simulink model "SGBMDisparity"  (R2021a)
settings: Solver=FixedStepDiscrete  StartTime=0.0  StopTime=simT  FixedStep=1  RelTol=1e-3
PreLoadFcn:
  | DL128 = Simulink.Variant('disparityLevels==128');
  | 
  | DLnot128 = Simulink.Variant('disparityLevels ~= 128');
  | 
  | disparityLevels = 64;
  | 
  | imgRowSize = 480;
  | 
  | imgColSize = 640;
  | 
  | P2 = 200; % Smoothness Penalty Large
  | P1 = 15;  % Smoothness Penalty Small
  | 
  | disparityFactor = 16;
  | 
  | uniquenessRatio = 5;
  | 
  | p = imgColSize - 1;
  | q = imgRowSize * imgColSize -1;
  | r = imgColSize - disparityLevels -1;
  | s = (imgRowSize*(imgColSize-disparityLevels))-1;
  | 
  | simT = 800*525
  | 
  | dtGain = 4;
InitFcn:
  | DL128 = Simulink.Variant('disparityLevels==128');
  | 
  | DLnot128 = Simulink.Variant('disparityLevels ~= 128');
  | 
  | img = imread(get_param('SGBMDisparity/stereoImage','FileName'));
  | 
  | [imgRowSize, imgColSize,chn] = size(img);
  | 
  | P2 = 200; % Smoothness Penalty Large
  | P1 = 15;  % Smoothness Penalty Small
  | 
  | disparityFactor = 16;
  | 
  | uniquenessRatio = str2num(get_param('SGBMDisparity/SGBMHDLAlgorithm/SGBMHDLAlgorithmWorker','UT'));
  | 
  | disparityLevels = str2num(get_param('SGBMDisparity/SGBMHDLAlgorithm/SGBMHDLAlgorithmWorker','DL'));
  | 
  | p = imgColSize - 1;
  | q = imgRowSize * imgColSize -1;
  | r = imgColSize - disparityLevels -1;
  | s = (imgRowSize*(imgColSize-disparityLevels))-1;
  | 
  | if imgRowSize == 720 && imgColSize == 1280
  | simT = 1650*750;
  | elseif imgRowSize == 540 && imgColSize == 960
  | simT = 1050*600;
  | elseif imgRowSize == 480 && imgColSize == 640
  | simT = 800*525;
  | end
  | 
  | %if imgRowSize == 720 && imgColSize == 1280
  | %dtGain = 2;
  | %elseif imgRowSize == 540 && imgColSize == 960
  | %dtGain = 2.6;
  | %elseif imgRowSize == 480 && imgColSize == 640
  | %dtGain = 4;
  | %end
  | 
  | dtGain = 8;
libraries: simulink x331, hdlsllib x113, visionhdlutilities x9, visionhdlio x2, visionsources x1
(part 3 of 6)

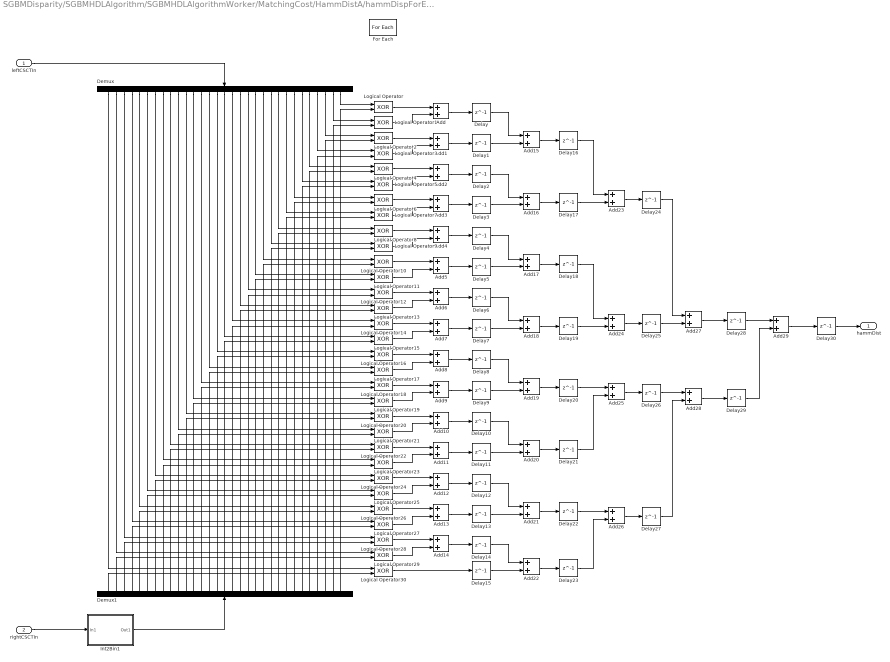
== system SGBMDisparity/SGBMHDLAlgorithm/SGBMHDLAlgorithmWorker/MatchingCost/HammDistA/hammDispForEach ==
  leftCSCTIn : Inport
  rightCSCTIn : Inport  Port=2  Partition=on  PartitionDimension=1  PartitionWidth=1  PartitionOffset=0
  Add{,1..14,22} (16 alike) : Sum  OutDataTypeStr=fixdt(0,2,0)
  Add{15..21,26} (8 alike) : Sum  OutDataTypeStr=fixdt(0,3,0)
  Add{23..25,28} (4 alike) : Sum  OutDataTypeStr=fixdt(0,4,0)
  Add27 : Sum  OutDataTypeStr=fixdt(0,5,0)
  Add29 : Sum  OutDataTypeStr=fixdt(0,5,0)
  Delay{,1..30} (31 alike) : Delay  DelayLength=1
  Demux : Demux  Outputs=31
  Demux1 : Demux  Outputs=31
  For Each : ForEach  DisableCoverage=on
  Int2Bin1 : Subsystem
  Logical Operator{,1..30} (31 alike) : Logic  Operator=XOR  OutDataTypeStr=boolean
  hammDist : Outport  ConcatenationDimension=1  VectorParamsAs1DForOutWhenUnconnected=off
  wires:
  Demux1/7 -> Logical Operator24/2
  Demux1/18 -> Logical Operator13/2
  Delay22/1 -> Add26/1
  Logical Operator19/1 -> Add9/2
  Demux/23 -> Logical Operator8/1
  Add26/1 -> Delay27/1
  Demux1/9 -> Logical Operator22/2
  Demux1/13 -> Logical Operator18/2
  Demux/10 -> Logical Operator21/1
  Demux/24 -> Logical Operator7/1
  Demux1/26 -> Logical Operator5/2
  Demux1/10 -> Logical Operator21/2
  Demux/14 -> Logical Operator17/1
  Demux1/17 -> Logical Operator14/2
  Delay18/1 -> Add24/1
  Demux1/15 -> Logical Operator16/2
  Demux1/11 -> Logical Operator20/2
  Demux/11 -> Logical Operator20/1
  Add27/1 -> Delay28/1
  Delay26/1 -> Add28/1
  Delay11/1 -> Add20/2
  Logical Operator13/1 -> Add6/2
  Add16/1 -> Delay17/1
  Add20/1 -> Delay21/1
  Demux/21 -> Logical Operator10/1
  Add18/1 -> Delay19/1
  Add23/1 -> Delay24/1
  Demux1/28 -> Logical Operator3/2
  Demux1/27 -> Logical Operator4/2
  Demux/26 -> Logical Operator5/1
  Demux/22 -> Logical Operator9/1
  Demux/25 -> Logical Operator6/1
  Demux/20 -> Logical Operator11/1
  Demux/8 -> Logical Operator23/1
  Demux1/29 -> Logical Operator2/2
  leftCSCTIn/1 -> Demux/1
  Logical Operator12/1 -> Add6/1
  Demux/19 -> Logical Operator12/1
  Add/1 -> Delay/1
  Demux/17 -> Logical Operator14/1
  Logical Operator22/1 -> Add11/1
  Demux/29 -> Logical Operator2/1
  Logical Operator16/1 -> Add8/1
  Logical Operator18/1 -> Add9/1
  Logical Operator17/1 -> Add8/2
  Logical Operator26/1 -> Add13/1
  Logical Operator24/1 -> Add12/1
  Logical Operator25/1 -> Add12/2
  Demux1/20 -> Logical Operator11/2
  Delay27/1 -> Add28/2
  Add13/1 -> Delay13/1
  Logical Operator4/1 -> Add2/1
  Logical Operator3/1 -> Add1/2
  Demux1/24 -> Logical Operator7/2
  Demux1/31 -> Logical Operator/2
  Logical Operator8/1 -> Add4/1
  Demux1/30 -> Logical Operator1/2
  Logical Operator5/1 -> Add2/2
  Logical Operator2/1 -> Add1/1
  Logical Operator7/1 -> Add3/2
  Logical Operator6/1 -> Add3/1
  Demux/30 -> Logical Operator1/1
  Delay29/1 -> Add29/2
  Demux1/25 -> Logical Operator6/2
  Logical Operator9/1 -> Add4/2
  Logical Operator14/1 -> Add7/1
  Demux/31 -> Logical Operator/1
  Delay21/1 -> Add25/2
  Delay24/1 -> Add27/1
  Delay23/1 -> Add26/2
  Logical Operator15/1 -> Add7/2
  Delay28/1 -> Add29/1
  Add28/1 -> Delay29/1
  Add22/1 -> Delay23/1
  Add25/1 -> Delay26/1
  Add24/1 -> Delay25/1
  Delay19/1 -> Add24/2
  Delay13/1 -> Add21/2
  rightCSCTIn/1 -> Int2Bin1/1(In1)
  Add1/1 -> Delay1/1
  Add17/1 -> Delay18/1
  Delay3/1 -> Add16/2
  Delay6/1 -> Add18/1
  Add12/1 -> Delay12/1
  Logical Operator30/1 -> Delay15/1
  Delay9/1 -> Add19/2
  Delay4/1 -> Add17/1
  Delay/1 -> Add15/1
  Add7/1 -> Delay7/1
  Add9/1 -> Delay9/1
  Add10/1 -> Delay10/1
  Add14/1 -> Delay14/1
  Add5/1 -> Delay5/1
  Add3/1 -> Delay3/1
  Logical Operator/1 -> Add/1
  Delay16/1 -> Add23/1
  Add29/1 -> Delay30/1
  Demux1/8 -> Logical Operator23/2
  Demux/4 -> Logical Operator27/1
  Demux1/5 -> Logical Operator26/2
  Demux/18 -> Logical Operator13/1
  Logical Operator1/1 -> Add/2
  Demux1/4 -> Logical Operator27/2
  Demux1/1 -> Logical Operator30/2
  Add2/1 -> Delay2/1
  Demux/16 -> Logical Operator15/1
  Demux1/12 -> Logical Operator19/2
  Demux1/2 -> Logical Operator29/2
  Delay12/1 -> Add21/1
  Demux/12 -> Logical Operator19/1
  Delay2/1 -> Add16/1
  Delay17/1 -> Add23/2
  Logical Operator27/1 -> Add13/2
  Delay20/1 -> Add25/1
  Demux/13 -> Logical Operator18/1
  Logical Operator28/1 -> Add14/1
  Add21/1 -> Delay22/1
  Demux/7 -> Logical Operator24/1
  Logical Operator21/1 -> Add10/2
  Demux/2 -> Logical Operator29/1
  Delay30/1 -> hammDist/1
  Demux1/19 -> Logical Operator12/2
  Delay15/1 -> Add22/2
  Demux/5 -> Logical Operator26/1
  Demux1/22 -> Logical Operator9/2
  Add6/1 -> Delay6/1
  Demux/28 -> Logical Operator3/1
  Delay7/1 -> Add18/2
  Logical Operator20/1 -> Add10/1
  Demux/6 -> Logical Operator25/1
  Logical Operator11/1 -> Add5/2
  Demux1/6 -> Logical Operator25/2
  Logical Operator23/1 -> Add11/2
  Add4/1 -> Delay4/1
  Delay8/1 -> Add19/1
  Add8/1 -> Delay8/1
  Add11/1 -> Delay11/1
  Demux/15 -> Logical Operator16/1
  Delay1/1 -> Add15/2
  Demux/9 -> Logical Operator22/1
  Demux/3 -> Logical Operator28/1
  Add15/1 -> Delay16/1
  Demux1/3 -> Logical Operator28/2
  Delay10/1 -> Add20/1
  Logical Operator29/1 -> Add14/2
  Demux1/23 -> Logical Operator8/2
  Delay14/1 -> Add22/1
  Delay5/1 -> Add17/2
  Demux1/21 -> Logical Operator10/2
  Demux/1 -> Logical Operator30/1
  Demux1/16 -> Logical Operator15/2
  Demux/27 -> Logical Operator4/1
  Demux1/14 -> Logical Operator17/2
  Add19/1 -> Delay20/1
  Logical Operator10/1 -> Add5/1
  Delay25/1 -> Add27/2
  Int2Bin1/1(Out1) -> Demux1/1

== system SGBMDisparity/SGBMHDLAlgorithm/SGBMHDLAlgorithmWorker/MatchingCost/HammDistA/pixelBusGenerator ==
  validIn : Inport
  Horizontal : hdlsllib/Sources/HDL Counter  CountType=Count limited  CountInit=0  CountStep=1  CountMax=hEnd  CountFromType=Initial value  CountFrom=0  CountResetPort=off  CountLoadPort=off  CountEnbPort=on  CountDirPort=off  CountHitOutputPort=off  CountDataType=Unsigned  CountWordLen=ceil(log2(hEnd))  CountFracLen=0  CountSampTime=1
  Logical Operator{3..6} (4 alike) : Logic  AllPortsSameDT=off  OutDataTypeStr=boolean
  Pixel Control Bus Creator : visionhdlutilities/Pixel Control Bus Creator
      settings: SourceProductBaseCode=VT
  Vertical : hdlsllib/Sources/HDL Counter  CountType=Count limited  CountInit=0  CountStep=1  CountMax=vEnd  CountFromType=Initial value  CountFrom=0  CountResetPort=off  CountLoadPort=off  CountEnbPort=on  CountDirPort=off  CountHitOutputPort=off  CountDataType=Unsigned  CountWordLen=ceil(log2(vEnd))  CountFracLen=0  CountSampTime=1
  hEnd : simulink/Logic and Bit Operations/Compare To Constant  relop===  const=hEnd  OutDataTypeStr=boolean
  hStart : simulink/Logic and Bit Operations/Compare To Constant  relop===  const=0  OutDataTypeStr=boolean
  vEnd : simulink/Logic and Bit Operations/Compare To Constant  relop===  const=vEnd  OutDataTypeStr=boolean
  vStart : simulink/Logic and Bit Operations/Compare To Constant  relop===  const=0  OutDataTypeStr=boolean
  busOut : Outport  VectorParamsAs1DForOutWhenUnconnected=off
  wires:
  validIn/1 -> Pixel Control Bus Creator/5, Vertical/1, Logical Operator4/1, Logical Operator5/1, Logical Operator6/1, Logical Operator3/1, Horizontal/1
  Horizontal/1 -> hEnd/1, hStart/1
  hEnd/1 -> Logical Operator4/2
  Vertical/1 -> vStart/1, vEnd/1
  vStart/1 -> Logical Operator5/2
  vEnd/1 -> Logical Operator6/2
  Logical Operator5/1 -> Pixel Control Bus Creator/3
  Logical Operator3/1 -> Pixel Control Bus Creator/1
  Logical Operator4/1 -> Pixel Control Bus Creator/2
  hStart/1 -> Logical Operator3/2
  Logical Operator6/1 -> Pixel Control Bus Creator/4
  Pixel Control Bus Creator/1 -> busOut/1

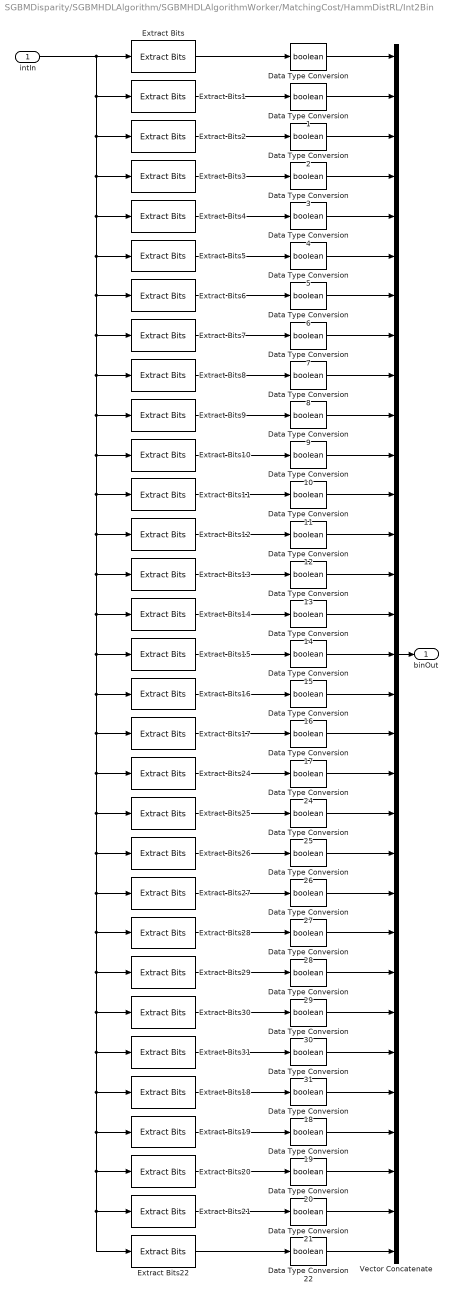
== system SGBMDisparity/SGBMHDLAlgorithm/SGBMHDLAlgorithmWorker/MatchingCost/HammDistRL/Int2Bin ==
  intIn : Inport
  Data Type Conversion{,1..22,24..31} (31 alike) : DataTypeConversion  OutDataTypeStr=boolean
  Extract Bits : simulink/Logic and Bit Operations/Extract Bits  bitsToExtract=Range of bits  numBits=8  bitIdxRange=[30]  outScalingMode=Treat bit field as an integer
  Extract Bits1 : simulink/Logic and Bit Operations/Extract Bits  bitsToExtract=Range of bits  numBits=8  bitIdxRange=[29]  outScalingMode=Treat bit field as an integer
  Extract Bits10 : simulink/Logic and Bit Operations/Extract Bits  bitsToExtract=Range of bits  numBits=8  bitIdxRange=[20]  outScalingMode=Preserve fixed-point scaling
  Extract Bits11 : simulink/Logic and Bit Operations/Extract Bits  bitsToExtract=Range of bits  numBits=8  bitIdxRange=[19]  outScalingMode=Preserve fixed-point scaling
  Extract Bits12 : simulink/Logic and Bit Operations/Extract Bits  bitsToExtract=Range of bits  numBits=8  bitIdxRange=[18]  outScalingMode=Preserve fixed-point scaling
  Extract Bits13 : simulink/Logic and Bit Operations/Extract Bits  bitsToExtract=Range of bits  numBits=8  bitIdxRange=[17]  outScalingMode=Preserve fixed-point scaling
  Extract Bits14 : simulink/Logic and Bit Operations/Extract Bits  bitsToExtract=Range of bits  numBits=8  bitIdxRange=[16]  outScalingMode=Preserve fixed-point scaling
  Extract Bits15 : simulink/Logic and Bit Operations/Extract Bits  bitsToExtract=Range of bits  numBits=8  bitIdxRange=[15]  outScalingMode=Preserve fixed-point scaling
  Extract Bits16 : simulink/Logic and Bit Operations/Extract Bits  bitsToExtract=Range of bits  numBits=8  bitIdxRange=[14]  outScalingMode=Preserve fixed-point scaling
  Extract Bits17 : simulink/Logic and Bit Operations/Extract Bits  bitsToExtract=Range of bits  numBits=8  bitIdxRange=[13]  outScalingMode=Preserve fixed-point scaling
  Extract Bits18 : simulink/Logic and Bit Operations/Extract Bits  bitsToExtract=Range of bits  numBits=8  bitIdxRange=[4]  outScalingMode=Preserve fixed-point scaling
  Extract Bits19 : simulink/Logic and Bit Operations/Extract Bits  bitsToExtract=Range of bits  numBits=8  bitIdxRange=[3]  outScalingMode=Preserve fixed-point scaling
  Extract Bits2 : simulink/Logic and Bit Operations/Extract Bits  bitsToExtract=Range of bits  numBits=8  bitIdxRange=[28]  outScalingMode=Treat bit field as an integer
  Extract Bits20 : simulink/Logic and Bit Operations/Extract Bits  bitsToExtract=Range of bits  numBits=8  bitIdxRange=[2]  outScalingMode=Preserve fixed-point scaling
  Extract Bits21 : simulink/Logic and Bit Operations/Extract Bits  bitsToExtract=Range of bits  numBits=8  bitIdxRange=[1]  outScalingMode=Preserve fixed-point scaling
  Extract Bits22 : simulink/Logic and Bit Operations/Extract Bits  bitsToExtract=Range of bits  numBits=8  bitIdxRange=[0]  outScalingMode=Preserve fixed-point scaling
  Extract Bits24 : simulink/Logic and Bit Operations/Extract Bits  bitsToExtract=Range of bits  numBits=8  bitIdxRange=[12]  outScalingMode=Preserve fixed-point scaling
  Extract Bits25 : simulink/Logic and Bit Operations/Extract Bits  bitsToExtract=Range of bits  numBits=8  bitIdxRange=[11]  outScalingMode=Preserve fixed-point scaling
  Extract Bits26 : simulink/Logic and Bit Operations/Extract Bits  bitsToExtract=Range of bits  numBits=8  bitIdxRange=[10]  outScalingMode=Preserve fixed-point scaling
  Extract Bits27 : simulink/Logic and Bit Operations/Extract Bits  bitsToExtract=Range of bits  numBits=8  bitIdxRange=[9]  outScalingMode=Preserve fixed-point scaling
  Extract Bits28 : simulink/Logic and Bit Operations/Extract Bits  bitsToExtract=Range of bits  numBits=8  bitIdxRange=[8]  outScalingMode=Preserve fixed-point scaling
  Extract Bits29 : simulink/Logic and Bit Operations/Extract Bits  bitsToExtract=Range of bits  numBits=8  bitIdxRange=[7]  outScalingMode=Preserve fixed-point scaling
  Extract Bits3 : simulink/Logic and Bit Operations/Extract Bits  bitsToExtract=Range of bits  numBits=8  bitIdxRange=[27]  outScalingMode=Treat bit field as an integer
  Extract Bits30 : simulink/Logic and Bit Operations/Extract Bits  bitsToExtract=Range of bits  numBits=8  bitIdxRange=[6]  outScalingMode=Preserve fixed-point scaling
  Extract Bits31 : simulink/Logic and Bit Operations/Extract Bits  bitsToExtract=Range of bits  numBits=8  bitIdxRange=[5]  outScalingMode=Preserve fixed-point scaling
  Extract Bits4 : simulink/Logic and Bit Operations/Extract Bits  bitsToExtract=Range of bits  numBits=8  bitIdxRange=[26]  outScalingMode=Treat bit field as an integer
  Extract Bits5 : simulink/Logic and Bit Operations/Extract Bits  bitsToExtract=Range of bits  numBits=8  bitIdxRange=[25]  outScalingMode=Treat bit field as an integer
  Extract Bits6 : simulink/Logic and Bit Operations/Extract Bits  bitsToExtract=Range of bits  numBits=8  bitIdxRange=[24]  outScalingMode=Treat bit field as an integer
  Extract Bits7 : simulink/Logic and Bit Operations/Extract Bits  bitsToExtract=Range of bits  numBits=8  bitIdxRange=[23]  outScalingMode=Treat bit field as an integer
  Extract Bits8 : simulink/Logic and Bit Operations/Extract Bits  bitsToExtract=Range of bits  numBits=8  bitIdxRange=[22]  outScalingMode=Preserve fixed-point scaling
  Extract Bits9 : simulink/Logic and Bit Operations/Extract Bits  bitsToExtract=Range of bits  numBits=8  bitIdxRange=[21]  outScalingMode=Preserve fixed-point scaling
  Vector Concatenate : Concatenate  NumInputs=31
  binOut : Outport  VectorParamsAs1DForOutWhenUnconnected=off
  wires:
  Extract Bits6/1 -> Data Type Conversion6/1
  Extract Bits8/1 -> Data Type Conversion8/1
  Extract Bits1/1 -> Data Type Conversion1/1
  Extract Bits2/1 -> Data Type Conversion2/1
  Extract Bits9/1 -> Data Type Conversion9/1
  Extract Bits10/1 -> Data Type Conversion10/1
  Extract Bits3/1 -> Data Type Conversion3/1
  Extract Bits4/1 -> Data Type Conversion4/1
  Extract Bits11/1 -> Data Type Conversion11/1
  Extract Bits12/1 -> Data Type Conversion12/1
  Extract Bits13/1 -> Data Type Conversion13/1
  Extract Bits/1 -> Data Type Conversion/1
  Extract Bits7/1 -> Data Type Conversion7/1
  Extract Bits5/1 -> Data Type Conversion5/1
  Extract Bits31/1 -> Data Type Conversion31/1
  Extract Bits26/1 -> Data Type Conversion26/1
  Extract Bits18/1 -> Data Type Conversion18/1
  Extract Bits14/1 -> Data Type Conversion14/1
  Extract Bits21/1 -> Data Type Conversion21/1
  Extract Bits16/1 -> Data Type Conversion16/1
  Extract Bits25/1 -> Data Type Conversion25/1
  Extract Bits27/1 -> Data Type Conversion27/1
  Extract Bits30/1 -> Data Type Conversion30/1
  Extract Bits20/1 -> Data Type Conversion20/1
  Extract Bits28/1 -> Data Type Conversion28/1
  Extract Bits22/1 -> Data Type Conversion22/1
  Extract Bits24/1 -> Data Type Conversion24/1
  Extract Bits19/1 -> Data Type Conversion19/1
  Extract Bits15/1 -> Data Type Conversion15/1
  Extract Bits17/1 -> Data Type Conversion17/1
  Extract Bits29/1 -> Data Type Conversion29/1
  Vector Concatenate/1 -> binOut/1
  intIn/1 -> Extract Bits/1, Extract Bits1/1, Extract Bits2/1, Extract Bits3/1, Extract Bits4/1, Extract Bits5/1, Extract Bits6/1, Extract Bits7/1, Extract Bits8/1, Extract Bits9/1, Extract Bits10/1, Extract Bits11/1, Extract Bits12/1, Extract Bits13/1, Extract Bits14/1, Extract Bits15/1, Extract Bits16/1, Extract Bits17/1, Extract Bits24/1, Extract Bits25/1, Extract Bits26/1, Extract Bits27/1, Extract Bits28/1, Extract Bits29/1, Extract Bits30/1, Extract Bits31/1, Extract Bits18/1, Extract Bits19/1, Extract Bits20/1, Extract Bits21/1, Extract Bits22/1
  Data Type Conversion/1 -> Vector Concatenate/1
  Data Type Conversion1/1 -> Vector Concatenate/2
  Data Type Conversion2/1 -> Vector Concatenate/3
  Data Type Conversion3/1 -> Vector Concatenate/4
  Data Type Conversion4/1 -> Vector Concatenate/5
  Data Type Conversion7/1 -> Vector Concatenate/8
  Data Type Conversion6/1 -> Vector Concatenate/7
  Data Type Conversion5/1 -> Vector Concatenate/6
  Data Type Conversion8/1 -> Vector Concatenate/9
  Data Type Conversion10/1 -> Vector Concatenate/11
  Data Type Conversion9/1 -> Vector Concatenate/10
  Data Type Conversion11/1 -> Vector Concatenate/12
  Data Type Conversion14/1 -> Vector Concatenate/15
  Data Type Conversion12/1 -> Vector Concatenate/13
  Data Type Conversion13/1 -> Vector Concatenate/14
  Data Type Conversion15/1 -> Vector Concatenate/16
  Data Type Conversion20/1 -> Vector Concatenate/29
  Data Type Conversion21/1 -> Vector Concatenate/30
  Data Type Conversion24/1 -> Vector Concatenate/19
  Data Type Conversion22/1 -> Vector Concatenate/31
  Data Type Conversion27/1 -> Vector Concatenate/22
  Data Type Conversion26/1 -> Vector Concatenate/21
  Data Type Conversion25/1 -> Vector Concatenate/20
  Data Type Conversion29/1 -> Vector Concatenate/24
  Data Type Conversion28/1 -> Vector Concatenate/23
  Data Type Conversion30/1 -> Vector Concatenate/25
  Data Type Conversion31/1 -> Vector Concatenate/26
  Data Type Conversion16/1 -> Vector Concatenate/17
  Data Type Conversion17/1 -> Vector Concatenate/18
  Data Type Conversion19/1 -> Vector Concatenate/28
  Data Type Conversion18/1 -> Vector Concatenate/27

== system SGBMDisparity/SGBMHDLAlgorithm/SGBMHDLAlgorithmWorker/MatchingCost/HammDistRL/enabledTappedDelay ==
  pixelIn : Inport
  Enable : EnablePort
  Tapped Delay : simulink/Discrete/Tapped Delay  vinit=0  samptime=-1  NumDelays=disparityLevels-1  DelayOrder=Oldest  includeCurrent=on
  pixelOut : Outport  InitialOutput=0  VectorParamsAs1DForOutWhenUnconnected=off
  wires:
  pixelIn/1 -> Tapped Delay/1
  Tapped Delay/1 -> pixelOut/1

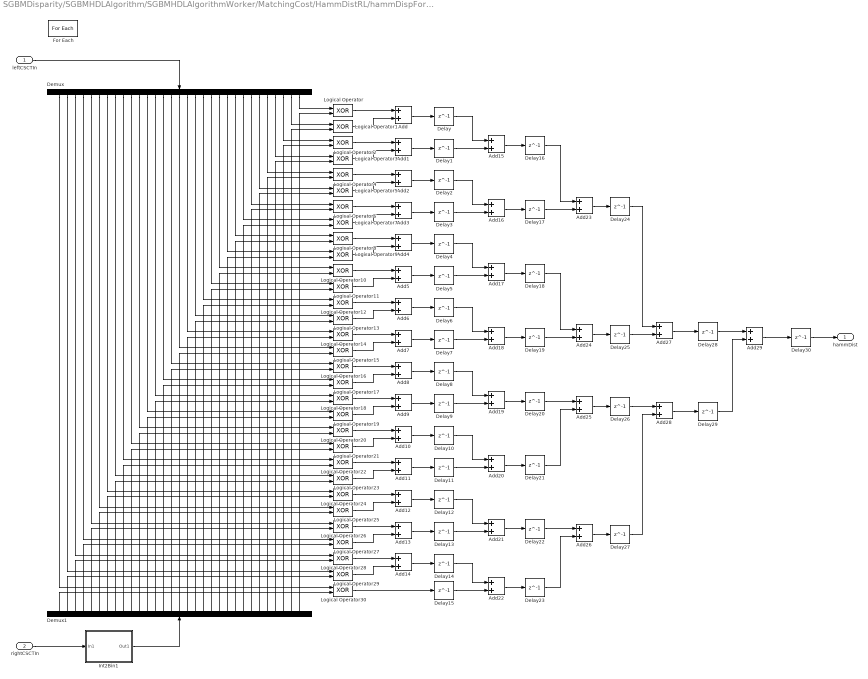
== system SGBMDisparity/SGBMHDLAlgorithm/SGBMHDLAlgorithmWorker/MatchingCost/HammDistRL/hammDispForEach ==
  leftCSCTIn : Inport
  rightCSCTIn : Inport  Port=2  Partition=on  PartitionDimension=1  PartitionWidth=1  PartitionOffset=0
  Add{,1..14,22} (16 alike) : Sum  OutDataTypeStr=fixdt(0,2,0)
  Add{15..21,26} (8 alike) : Sum  OutDataTypeStr=fixdt(0,3,0)
  Add{23..25,28} (4 alike) : Sum  OutDataTypeStr=fixdt(0,4,0)
  Add27 : Sum  OutDataTypeStr=fixdt(0,5,0)
  Add29 : Sum  OutDataTypeStr=fixdt(0,5,0)
  Delay{,1..30} (31 alike) : Delay  DelayLength=1
  Demux : Demux  Outputs=31
  Demux1 : Demux  Outputs=31
  For Each : ForEach  DisableCoverage=on
  Int2Bin1 : Subsystem
  Logical Operator{,1..30} (31 alike) : Logic  Operator=XOR  OutDataTypeStr=boolean
  hammDist : Outport  ConcatenationDimension=1  VectorParamsAs1DForOutWhenUnconnected=off
  wires:
  Demux1/7 -> Logical Operator24/2
  Demux1/18 -> Logical Operator13/2
  Delay22/1 -> Add26/1
  Logical Operator19/1 -> Add9/2
  Demux/23 -> Logical Operator8/1
  Add26/1 -> Delay27/1
  Demux1/9 -> Logical Operator22/2
  Demux1/13 -> Logical Operator18/2
  Demux/10 -> Logical Operator21/1
  Demux/24 -> Logical Operator7/1
  Demux1/26 -> Logical Operator5/2
  Demux1/10 -> Logical Operator21/2
  Demux/14 -> Logical Operator17/1
  Demux1/17 -> Logical Operator14/2
  Delay18/1 -> Add24/1
  Demux1/15 -> Logical Operator16/2
  Demux1/11 -> Logical Operator20/2
  Demux/11 -> Logical Operator20/1
  Add27/1 -> Delay28/1
  Delay26/1 -> Add28/1
  Delay11/1 -> Add20/2
  Logical Operator13/1 -> Add6/2
  Add16/1 -> Delay17/1
  Add20/1 -> Delay21/1
  Demux/21 -> Logical Operator10/1
  Add18/1 -> Delay19/1
  Add23/1 -> Delay24/1
  Demux1/28 -> Logical Operator3/2
  Demux1/27 -> Logical Operator4/2
  Demux/26 -> Logical Operator5/1
  Demux/22 -> Logical Operator9/1
  Demux/25 -> Logical Operator6/1
  Demux/20 -> Logical Operator11/1
  Demux/8 -> Logical Operator23/1
  Demux1/29 -> Logical Operator2/2
  leftCSCTIn/1 -> Demux/1
  Logical Operator12/1 -> Add6/1
  Demux/19 -> Logical Operator12/1
  Add/1 -> Delay/1
  Demux/17 -> Logical Operator14/1
  Logical Operator22/1 -> Add11/1
  Demux/29 -> Logical Operator2/1
  Logical Operator16/1 -> Add8/1
  Logical Operator18/1 -> Add9/1
  Logical Operator17/1 -> Add8/2
  Logical Operator26/1 -> Add13/1
  Logical Operator24/1 -> Add12/1
  Logical Operator25/1 -> Add12/2
  Demux1/20 -> Logical Operator11/2
  Delay27/1 -> Add28/2
  Add13/1 -> Delay13/1
  Logical Operator4/1 -> Add2/1
  Logical Operator3/1 -> Add1/2
  Demux1/24 -> Logical Operator7/2
  Demux1/31 -> Logical Operator/2
  Logical Operator8/1 -> Add4/1
  Demux1/30 -> Logical Operator1/2
  Logical Operator5/1 -> Add2/2
  Logical Operator2/1 -> Add1/1
  Logical Operator7/1 -> Add3/2
  Logical Operator6/1 -> Add3/1
  Demux/30 -> Logical Operator1/1
  Delay29/1 -> Add29/2
  Demux1/25 -> Logical Operator6/2
  Logical Operator9/1 -> Add4/2
  Logical Operator14/1 -> Add7/1
  Demux/31 -> Logical Operator/1
  Delay21/1 -> Add25/2
  Delay24/1 -> Add27/1
  Delay23/1 -> Add26/2
  Logical Operator15/1 -> Add7/2
  Delay28/1 -> Add29/1
  Add28/1 -> Delay29/1
  Add22/1 -> Delay23/1
  Add25/1 -> Delay26/1
  Add24/1 -> Delay25/1
  Delay19/1 -> Add24/2
  Delay13/1 -> Add21/2
  rightCSCTIn/1 -> Int2Bin1/1(In1)
  Add1/1 -> Delay1/1
  Add17/1 -> Delay18/1
  Delay3/1 -> Add16/2
  Delay6/1 -> Add18/1
  Add12/1 -> Delay12/1
  Logical Operator30/1 -> Delay15/1
  Delay9/1 -> Add19/2
  Delay4/1 -> Add17/1
  Delay/1 -> Add15/1
  Add7/1 -> Delay7/1
  Add9/1 -> Delay9/1
  Add10/1 -> Delay10/1
  Add14/1 -> Delay14/1
  Add5/1 -> Delay5/1
  Add3/1 -> Delay3/1
  Logical Operator/1 -> Add/1
  Delay16/1 -> Add23/1
  Add29/1 -> Delay30/1
  Demux1/8 -> Logical Operator23/2
  Demux/4 -> Logical Operator27/1
  Demux1/5 -> Logical Operator26/2
  Demux/18 -> Logical Operator13/1
  Logical Operator1/1 -> Add/2
  Demux1/4 -> Logical Operator27/2
  Demux1/1 -> Logical Operator30/2
  Add2/1 -> Delay2/1
  Demux/16 -> Logical Operator15/1
  Demux1/12 -> Logical Operator19/2
  Demux1/2 -> Logical Operator29/2
  Delay12/1 -> Add21/1
  Demux/12 -> Logical Operator19/1
  Delay2/1 -> Add16/1
  Delay17/1 -> Add23/2
  Logical Operator27/1 -> Add13/2
  Delay20/1 -> Add25/1
  Demux/13 -> Logical Operator18/1
  Logical Operator28/1 -> Add14/1
  Add21/1 -> Delay22/1
  Demux/7 -> Logical Operator24/1
  Logical Operator21/1 -> Add10/2
  Demux/2 -> Logical Operator29/1
  Delay30/1 -> hammDist/1
  Demux1/19 -> Logical Operator12/2
  Delay15/1 -> Add22/2
  Demux/5 -> Logical Operator26/1
  Demux1/22 -> Logical Operator9/2
  Add6/1 -> Delay6/1
  Demux/28 -> Logical Operator3/1
  Delay7/1 -> Add18/2
  Logical Operator20/1 -> Add10/1
  Demux/6 -> Logical Operator25/1
  Logical Operator11/1 -> Add5/2
  Demux1/6 -> Logical Operator25/2
  Logical Operator23/1 -> Add11/2
  Add4/1 -> Delay4/1
  Delay8/1 -> Add19/1
  Add8/1 -> Delay8/1
  Add11/1 -> Delay11/1
  Demux/15 -> Logical Operator16/1
  Delay1/1 -> Add15/2
  Demux/9 -> Logical Operator22/1
  Demux/3 -> Logical Operator28/1
  Add15/1 -> Delay16/1
  Demux1/3 -> Logical Operator28/2
  Delay10/1 -> Add20/1
  Logical Operator29/1 -> Add14/2
  Demux1/23 -> Logical Operator8/2
  Delay14/1 -> Add22/1
  Delay5/1 -> Add17/2
  Demux1/21 -> Logical Operator10/2
  Demux/1 -> Logical Operator30/1
  Demux1/16 -> Logical Operator15/2
  Demux/27 -> Logical Operator4/1
  Demux1/14 -> Logical Operator17/2
  Add19/1 -> Delay20/1
  Logical Operator10/1 -> Add5/1
  Delay25/1 -> Add27/2
  Int2Bin1/1(Out1) -> Demux1/1

== system SGBMDisparity/SGBMHDLAlgorithm/SGBMHDLAlgorithmWorker/MatchingCost/HammDistRL/inverseRowLeft ==
  leftIn : Inport
  leftBus : Inport  Port=2
  Bus Selector : BusSelector  OutputSignals=valid,hStart,hEnd,vStart
  Compare To Constant : simulink/Logic and Bit Operations/Compare To Constant  relop===  const=1  OutDataTypeStr=boolean
  Compare To Constant1 : simulink/Logic and Bit Operations/Compare To Constant  relop===  const=1  OutDataTypeStr=boolean
  Compare To Constant3 : simulink/Logic and Bit Operations/Compare To Constant  relop===  const=1  OutDataTypeStr=boolean
  Compare To Constant4 : simulink/Logic and Bit Operations/Compare To Constant  relop===  const=imgColSize-1  OutDataTypeStr=boolean
  Constant : Constant  Value=0  OutDataTypeStr=boolean  SampleTime=-1
  Constant1 : Constant  Value=0  OutDataTypeStr=boolean  SampleTime=-1
  Delay{1..8} (8 alike) : Delay  DelayLength=1
  HDL Counter : hdlsllib/Sources/HDL Counter  CountType=Count limited  CountInit=0  CountStep=1  CountMax=imgColSize-1  CountFromType=Initial value  CountFrom=0  CountResetPort=on  CountLoadPort=off  CountEnbPort=on  CountDirPort=off  CountHitOutputPort=off  CountDataType=Unsigned  CountWordLen=ceil(log2(imgColSize-1))  CountFracLen=0  CountSampTime=1
  HDL Counter1 : hdlsllib/Sources/HDL Counter  CountType=Count limited  CountInit=imgColSize-1  CountStep=1  CountMax=0  CountFromType=Initial value  CountFrom=imgColSize-1  CountResetPort=on  CountLoadPort=off  CountEnbPort=on  CountDirPort=on  CountHitOutputPort=off  CountDataType=Unsigned  CountWordLen=ceil(log2(imgColSize-1))  CountFracLen=0  CountSampTime=1
  HDL Counter2 : hdlsllib/Sources/HDL Counter  CountType=Count limited  CountInit=0  CountStep=1  CountMax=1  CountFromType=Initial value  CountFrom=0  CountResetPort=on  CountLoadPort=off  CountEnbPort=on  CountDirPort=off  CountHitOutputPort=off  CountDataType=Unsigned  CountWordLen=1  CountFracLen=0  CountSampTime=1
  HDL Counter3 : hdlsllib/Sources/HDL Counter  CountType=Count limited  CountInit=imgColSize-1  CountStep=1  CountMax=0  CountFromType=Initial value  CountFrom=imgColSize-1  CountResetPort=on  CountLoadPort=off  CountEnbPort=on  CountDirPort=on  CountHitOutputPort=off  CountDataType=Unsigned  CountWordLen=ceil(log2(imgColSize-1))  CountFracLen=0  CountSampTime=1
  HDL Counter4 : hdlsllib/Sources/HDL Counter  CountType=Count limited  CountInit=0  CountStep=1  CountMax=imgColSize-1  CountFromType=Initial value  CountFrom=0  CountResetPort=on  CountLoadPort=off  CountEnbPort=on  CountDirPort=off  CountHitOutputPort=off  CountDataType=Unsigned  CountWordLen=ceil(log2(imgColSize-1))  CountFracLen=0  CountSampTime=1
  HDL Counter5 : hdlsllib/Sources/HDL Counter  CountType=Count limited  CountInit=0  CountStep=1  CountMax=1  CountFromType=Initial value  CountFrom=0  CountResetPort=on  CountLoadPort=off  CountEnbPort=on  CountDirPort=off  CountHitOutputPort=off  CountDataType=Unsigned  CountWordLen=1  CountFracLen=0  CountSampTime=1
  HDL Counter6 : hdlsllib/Sources/HDL Counter  CountType=Count limited  CountInit=0  CountStep=1  CountMax=imgColSize+1  CountFromType=Initial value  CountFrom=0  CountResetPort=on  CountLoadPort=off  CountEnbPort=on  CountDirPort=off  CountHitOutputPort=off  CountDataType=Unsigned  CountWordLen=ceil(log2(imgColSize))  CountFracLen=0  CountSampTime=1
  HDL Counter7 : hdlsllib/Sources/HDL Counter  CountType=Count limited  CountInit=0  CountStep=1  CountMax=1  CountFromType=Initial value  CountFrom=0  CountResetPort=on  CountLoadPort=off  CountEnbPort=on  CountDirPort=off  CountHitOutputPort=off  CountDataType=Unsigned  CountWordLen=2  CountFracLen=0  CountSampTime=1
  Logical Operator : Logic  AllPortsSameDT=off  OutDataTypeStr=boolean
  Logical Operator1 : Logic  Operator=OR  AllPortsSameDT=off  OutDataTypeStr=boolean
  Rd_En : simulink/Logic and Bit Operations/Compare To Constant  relop=<=  const=imgColSize-1  OutDataTypeStr=boolean
  Simple Dual Port RAM : hdlsllib/HDL RAMs/Simple Dual Port RAM  ram_size=ceil(log2(imgColSize-1))
      settings: SourceProductBaseCode=SL
  Switch : Switch  Criteria=u2 ~= 0
  Switch1 : Switch  Criteria=u2 ~= 0
  leftValid : Outport  VectorParamsAs1DForOutWhenUnconnected=off
  leftOut : Outport  Port=2  VectorParamsAs1DForOutWhenUnconnected=off
  leftvStart : Outport  Port=3  VectorParamsAs1DForOutWhenUnconnected=off
  wires:
  Logical Operator/1 -> Delay7/1, HDL Counter4/2, HDL Counter3/2
  Compare To Constant4/1 -> Logical Operator1/2, HDL Counter6/1
  HDL Counter5/1 -> Compare To Constant1/1
  Switch1/1 -> Simple Dual Port RAM/4
  Compare To Constant3/1 -> Logical Operator/1, HDL Counter6/2
  HDL Counter2/1 -> Compare To Constant/1
  Constant1/1 -> HDL Counter3/3
  Bus Selector/2 -> Delay6/1  "<hStart>"
  HDL Counter4/1 -> Switch1/3
  Compare To Constant1/1 -> Switch1/2
  HDL Counter3/1 -> Switch1/1
  HDL Counter6/1 -> Rd_En/1, Compare To Constant4/1
  Delay2/1 -> Simple Dual Port RAM/1
  HDL Counter/1 -> Switch/1
  Constant/1 -> HDL Counter1/3
  HDL Counter1/1 -> Switch/3
  Delay1/1 -> Simple Dual Port RAM/3, HDL Counter1/2, HDL Counter/2
  Bus Selector/3 -> Delay8/1  "<hEnd>"
  Switch/1 -> Simple Dual Port RAM/2
  Delay7/1 -> leftValid/1
  Bus Selector/1 -> Delay5/1  "<valid>"
  HDL Counter7/1 -> Compare To Constant3/1
  Delay3/1 -> HDL Counter7/2, HDL Counter5/2
  Rd_En/1 -> Logical Operator/2
  Compare To Constant/1 -> Switch/2
  Simple Dual Port RAM/1 -> leftOut/1
  leftIn/1 -> Delay4/1
  leftBus/1 -> Bus Selector/1
  Logical Operator1/1 -> HDL Counter7/1
  Bus Selector/4 -> HDL Counter/1, HDL Counter1/1, HDL Counter4/1, HDL Counter3/1, HDL Counter5/1, leftvStart/1, Logical Operator1/1, HDL Counter2/1  "<vStart>"
  Delay4/1 -> Delay2/1
  Delay5/1 -> Delay1/1
  Delay6/1 -> HDL Counter2/2
  Delay8/1 -> Delay3/1

== system SGBMDisparity/SGBMHDLAlgorithm/SGBMHDLAlgorithmWorker/MatchingCost/HammDistRL/inverseRowLeft1 ==
  rightIn : Inport
  rightBus : Inport  Port=2
  Bus Selector : BusSelector  OutputSignals=valid,hStart,hEnd,vStart
  Compare To Constant : simulink/Logic and Bit Operations/Compare To Constant  relop===  const=1  OutDataTypeStr=boolean
  Compare To Constant1 : simulink/Logic and Bit Operations/Compare To Constant  relop===  const=1  OutDataTypeStr=boolean
  Compare To Constant3 : simulink/Logic and Bit Operations/Compare To Constant  relop===  const=1  OutDataTypeStr=boolean
  Compare To Constant4 : simulink/Logic and Bit Operations/Compare To Constant  relop===  const=imgColSize-1  OutDataTypeStr=boolean
  Constant : Constant  Value=0  OutDataTypeStr=boolean  SampleTime=-1
  Constant1 : Constant  Value=0  OutDataTypeStr=boolean  SampleTime=-1
  Delay{1..8} (8 alike) : Delay  DelayLength=1
  HDL Counter : hdlsllib/Sources/HDL Counter  CountType=Count limited  CountInit=0  CountStep=1  CountMax=imgColSize-1  CountFromType=Initial value  CountFrom=0  CountResetPort=on  CountLoadPort=off  CountEnbPort=on  CountDirPort=off  CountHitOutputPort=off  CountDataType=Unsigned  CountWordLen=ceil(log2(imgColSize-1))  CountFracLen=0  CountSampTime=1
  HDL Counter1 : hdlsllib/Sources/HDL Counter  CountType=Count limited  CountInit=imgColSize-1  CountStep=1  CountMax=0  CountFromType=Initial value  CountFrom=imgColSize-1  CountResetPort=on  CountLoadPort=off  CountEnbPort=on  CountDirPort=on  CountHitOutputPort=off  CountDataType=Unsigned  CountWordLen=ceil(log2(imgColSize-1))  CountFracLen=0  CountSampTime=1
  HDL Counter2 : hdlsllib/Sources/HDL Counter  CountType=Count limited  CountInit=0  CountStep=1  CountMax=1  CountFromType=Initial value  CountFrom=0  CountResetPort=on  CountLoadPort=off  CountEnbPort=on  CountDirPort=off  CountHitOutputPort=off  CountDataType=Unsigned  CountWordLen=1  CountFracLen=0  CountSampTime=1
  HDL Counter3 : hdlsllib/Sources/HDL Counter  CountType=Count limited  CountInit=imgColSize-1  CountStep=1  CountMax=0  CountFromType=Initial value  CountFrom=imgColSize-1  CountResetPort=on  CountLoadPort=off  CountEnbPort=on  CountDirPort=on  CountHitOutputPort=off  CountDataType=Unsigned  CountWordLen=ceil(log2(imgColSize-1))  CountFracLen=0  CountSampTime=1
  HDL Counter4 : hdlsllib/Sources/HDL Counter  CountType=Count limited  CountInit=0  CountStep=1  CountMax=imgColSize-1  CountFromType=Initial value  CountFrom=0  CountResetPort=on  CountLoadPort=off  CountEnbPort=on  CountDirPort=off  CountHitOutputPort=off  CountDataType=Unsigned  CountWordLen=ceil(log2(imgColSize-1))  CountFracLen=0  CountSampTime=1
  HDL Counter5 : hdlsllib/Sources/HDL Counter  CountType=Count limited  CountInit=0  CountStep=1  CountMax=1  CountFromType=Initial value  CountFrom=0  CountResetPort=on  CountLoadPort=off  CountEnbPort=on  CountDirPort=off  CountHitOutputPort=off  CountDataType=Unsigned  CountWordLen=1  CountFracLen=0  CountSampTime=1
  HDL Counter6 : hdlsllib/Sources/HDL Counter  CountType=Count limited  CountInit=0  CountStep=1  CountMax=imgColSize+1  CountFromType=Initial value  CountFrom=0  CountResetPort=on  CountLoadPort=off  CountEnbPort=on  CountDirPort=off  CountHitOutputPort=off  CountDataType=Unsigned  CountWordLen=ceil(log2(imgColSize))  CountFracLen=0  CountSampTime=1
  HDL Counter7 : hdlsllib/Sources/HDL Counter  CountType=Count limited  CountInit=0  CountStep=1  CountMax=1  CountFromType=Initial value  CountFrom=0  CountResetPort=on  CountLoadPort=off  CountEnbPort=on  CountDirPort=off  CountHitOutputPort=off  CountDataType=Unsigned  CountWordLen=2  CountFracLen=0  CountSampTime=1
  Logical Operator : Logic  AllPortsSameDT=off  OutDataTypeStr=boolean
  Logical Operator1 : Logic  Operator=OR  AllPortsSameDT=off  OutDataTypeStr=boolean
  Rd_En : simulink/Logic and Bit Operations/Compare To Constant  relop=<=  const=imgColSize-1  OutDataTypeStr=boolean
  Simple Dual Port RAM : hdlsllib/HDL RAMs/Simple Dual Port RAM  ram_size=ceil(log2(imgColSize-1))
      settings: SourceProductBaseCode=SL
  Switch : Switch  Criteria=u2 ~= 0
  Switch1 : Switch  Criteria=u2 ~= 0
  rightValid : Outport  VectorParamsAs1DForOutWhenUnconnected=off
  rightOut : Outport  Port=2  VectorParamsAs1DForOutWhenUnconnected=off
  rightvStart : Outport  Port=3  VectorParamsAs1DForOutWhenUnconnected=off
  wires:
  Logical Operator/1 -> Delay7/1, HDL Counter4/2, HDL Counter3/2
  Compare To Constant4/1 -> Logical Operator1/2, HDL Counter6/1
  HDL Counter5/1 -> Compare To Constant1/1
  Switch1/1 -> Simple Dual Port RAM/4
  Compare To Constant3/1 -> Logical Operator/1, HDL Counter6/2
  HDL Counter2/1 -> Compare To Constant/1
  Constant1/1 -> HDL Counter3/3
  Bus Selector/2 -> Delay6/1  "<hStart>"
  HDL Counter4/1 -> Switch1/3
  Compare To Constant1/1 -> Switch1/2
  HDL Counter3/1 -> Switch1/1
  HDL Counter6/1 -> Rd_En/1, Compare To Constant4/1
  Delay2/1 -> Simple Dual Port RAM/1
  HDL Counter/1 -> Switch/1
  Constant/1 -> HDL Counter1/3
  HDL Counter1/1 -> Switch/3
  Delay1/1 -> Simple Dual Port RAM/3, HDL Counter1/2, HDL Counter/2
  Bus Selector/3 -> Delay8/1  "<hEnd>"
  Switch/1 -> Simple Dual Port RAM/2
  Delay7/1 -> rightValid/1
  Bus Selector/1 -> Delay5/1  "<valid>"
  HDL Counter7/1 -> Compare To Constant3/1
  Delay3/1 -> HDL Counter7/2, HDL Counter5/2
  Rd_En/1 -> Logical Operator/2
  Compare To Constant/1 -> Switch/2
  Simple Dual Port RAM/1 -> rightOut/1
  rightIn/1 -> Delay4/1
  rightBus/1 -> Bus Selector/1
  Logical Operator1/1 -> HDL Counter7/1
  Bus Selector/4 -> HDL Counter/1, HDL Counter1/1, HDL Counter4/1, HDL Counter3/1, HDL Counter5/1, rightvStart/1, Logical Operator1/1, HDL Counter2/1  "<vStart>"
  Delay4/1 -> Delay2/1
  Delay5/1 -> Delay1/1
  Delay6/1 -> HDL Counter2/2
  Delay8/1 -> Delay3/1

== system SGBMDisparity/SGBMHDLAlgorithm/SGBMHDLAlgorithmWorker/MatchingCost/HammDistRL/pixelBusGenerator ==
  validIn : Inport
  Horizontal : hdlsllib/Sources/HDL Counter  CountType=Count limited  CountInit=0  CountStep=1  CountMax=hEnd  CountFromType=Initial value  CountFrom=0  CountResetPort=off  CountLoadPort=off  CountEnbPort=on  CountDirPort=off  CountHitOutputPort=off  CountDataType=Unsigned  CountWordLen=ceil(log2(hEnd))  CountFracLen=0  CountSampTime=1
  Logical Operator{3..6} (4 alike) : Logic  AllPortsSameDT=off  OutDataTypeStr=boolean
  Pixel Control Bus Creator : visionhdlutilities/Pixel Control Bus Creator
      settings: SourceProductBaseCode=VT
  Vertical : hdlsllib/Sources/HDL Counter  CountType=Count limited  CountInit=0  CountStep=1  CountMax=vEnd  CountFromType=Initial value  CountFrom=0  CountResetPort=off  CountLoadPort=off  CountEnbPort=on  CountDirPort=off  CountHitOutputPort=off  CountDataType=Unsigned  CountWordLen=ceil(log2(vEnd))  CountFracLen=0  CountSampTime=1
  hEnd : simulink/Logic and Bit Operations/Compare To Constant  relop===  const=hEnd  OutDataTypeStr=boolean
  hStart : simulink/Logic and Bit Operations/Compare To Constant  relop===  const=0  OutDataTypeStr=boolean
  vEnd : simulink/Logic and Bit Operations/Compare To Constant  relop===  const=vEnd  OutDataTypeStr=boolean
  vStart : simulink/Logic and Bit Operations/Compare To Constant  relop===  const=0  OutDataTypeStr=boolean
  busOut : Outport  VectorParamsAs1DForOutWhenUnconnected=off
  wires:
  validIn/1 -> Pixel Control Bus Creator/5, Vertical/1, Logical Operator4/1, Logical Operator5/1, Logical Operator6/1, Logical Operator3/1, Horizontal/1
  Horizontal/1 -> hEnd/1, hStart/1
  hEnd/1 -> Logical Operator4/2
  Vertical/1 -> vStart/1, vEnd/1
  vStart/1 -> Logical Operator5/2
  vEnd/1 -> Logical Operator6/2
  Logical Operator5/1 -> Pixel Control Bus Creator/3
  Logical Operator3/1 -> Pixel Control Bus Creator/1
  Logical Operator4/1 -> Pixel Control Bus Creator/2
  hStart/1 -> Logical Operator3/2
  Logical Operator6/1 -> Pixel Control Bus Creator/4
  Pixel Control Bus Creator/1 -> busOut/1

== system SGBMDisparity/SGBMHDLAlgorithm/SGBMHDLAlgorithmWorker/PostProcessing/Interpolation/Division ==
  Dividend : Inport
  Divisor : Inport  Port=2
  QuoRem : Subsystem
  Rem2Bin : Subsystem
  res : Outport  VectorParamsAs1DForOutWhenUnconnected=off
  wires:
  Rem2Bin/1(val) -> res/1
  Divisor/1 -> QuoRem/2(Divisor)
  QuoRem/2(Div) -> Rem2Bin/2(Div)
  Dividend/1 -> QuoRem/1(Dividend)
  QuoRem/1(Quo) -> Rem2Bin/1(Quo)
  QuoRem/3(Rem) -> Rem2Bin/3(Rem)
